simulink model "kadai2"  (R2024a)
settings: Solver=VariableStepAuto  StartTime=0.0  StopTime=10.0  RelTol=1e-3
values from neighbouring files (symbols this model uses):
  e0 = 24.6    [contstants.m]
  g = 9.8    [contstants.m]
  i0 = 1.21    [contstants.m]
  k = 2.9e-4    (= 0.00029)    [contstants.m]
  Ki = 2*k*i0/x0.^2    [contstants.m]
  Kx = 2*k*i0.^2/x0.^3    [contstants.m]
  L = 0.51    [contstants.m]
  M = 1.75    [contstants.m]
  R = 23.2    [contstants.m]
  s = tf('s')    [rlocus.m]
  x0 = 5.0e-3    (= 0.005)    [contstants.m]
libraries: slctrl_linear x2
settings Model: Creator=thistle  LastModifiedBy=thistle

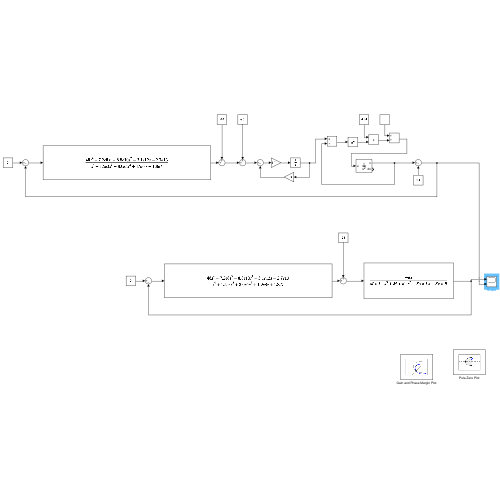
[thumbnail: Simulink's stored preview of the top-level diagram]
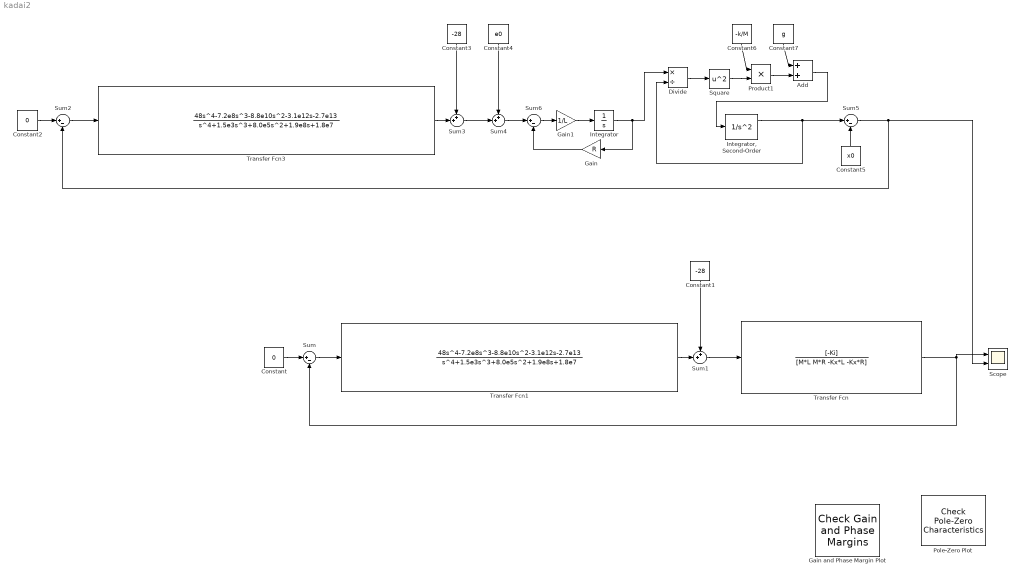
== system kadai2 ==
  Add : Sum
  Constant : Constant  Value=0
  Constant1 : Constant  Value=-28
  Constant2 : Constant  Value=0
  Constant3 : Constant  Value=-28
  Constant4 : Constant  Value=e0
  Constant5 : Constant  Value=x0
  Constant6 : Constant  Value=-k/M
  Constant7 : Constant  Value=g
  Divide : Product  Inputs=*/
  Gain : Gain  Gain=R
  Gain and Phase Margin Plot : slctrl_linear/Check Gain and Phase Margins  InstantiateOnLoad=on  SaveOperatingPoints=off  LinearizationIOs={'/Transfer Fcn', 1, 'out', 'on', '';'/Constant', 1, 'in', 'on', ''}  LinearizeAt=SnapshotTimes  SnapshotTimes=[0]  TriggerType=rising  SampleTime=auto  RateConversionMethod=zoh  PreWarpFreq=10  UseExactDelayModel=off  UseFullBlockNameLabels=off  UseBusSignalLabels=off  enabled=on  stopWhenAssertionFail=off  export=off  ViewDlgPos=[565.666666666667 151 510 390]  LaunchViewOnOpen=off  OpenViewOnLoad=off  FrequencyUnits=rad/s  MagnitudeUnits=dB  PhaseUnits=deg  TimeUnits=seconds  EnableMargins=off  GainMargin=[]  PhaseMargin=[]  PlotType=nyquist  FeedbackSign=-1
      settings: LibrarySourceBlock=slctrlblks/Linear Analysis Plots/Gain and Phase Margin Plot  SaveToWorkspace=off  SaveName=sys
  Gain1 : Gain  Gain=1/L
  Integrator : Integrator  InitialCondition=i0
  "Integrator, Second-Order" : SecondOrderIntegrator  ICX=x0
  Pole-Zero Plot : slctrl_linear/Check Pole-Zero Characteristics  InstantiateOnLoad=on  SaveOperatingPoints=off  LinearizationIOs={'/Constant', 1, 'in', 'on', '';'/Transfer Fcn', 1, 'out', 'on', ''}  LinearizeAt=SnapshotTimes  SnapshotTimes=[0]  TriggerType=rising  SampleTime=auto  RateConversionMethod=zoh  PreWarpFreq=10  UseExactDelayModel=off  UseFullBlockNameLabels=off  UseBusSignalLabels=off  enabled=on  stopWhenAssertionFail=off  export=off  ViewDlgPos=[1 1 1280 647.333333333333]  LaunchViewOnOpen=off  OpenViewOnLoad=off  FrequencyUnits=rad/s  MagnitudeUnits=dB  PhaseUnits=deg  TimeUnits=seconds  EnableSettlingTime=off  SettlingTime=[]  EnablePercentOvershoot=off  PercentOvershoot=[]  EnableDampingRatio=off  DampingRatio=[]  EnableNaturalFrequency=off  NaturalFrequencyBound=>=  NaturalFrequency=[]
      settings: LibrarySourceBlock=slctrlblks/Linear Analysis Plots/Pole-Zero Plot  SaveToWorkspace=off  SaveName=sys
  Product1 : Product
  Scope : Scope  NumInputPorts=2
  Square : Math  Operator=square
  Sum{,2,5..6} (4 alike) : Sum  Inputs=|+-
  Sum1 : Sum  Inputs=++|
  Sum3 : Sum  Inputs=++|
  Sum4 : Sum  Inputs=++|
  Transfer Fcn : TransferFcn  Numerator=[-Ki]  Denominator=[M*L M*R -Kx*L -Kx*R]
  Transfer Fcn1 : TransferFcn  Numerator=[48 -7.2e8 -8.8e10 -3.1e12 -2.7e13]  Denominator=[1 1.5e3 8.0e5 1.9e8 1.8e7]
  Transfer Fcn3 : TransferFcn  Numerator=[48 -7.2e8 -8.8e10 -3.1e12 -2.7e13]  Denominator=[1 1.5e3 8.0e5 1.9e8 1.8e7]
  wires:
  Constant/1 -> Sum/1
  Sum/1 -> Transfer Fcn1/1
  Transfer Fcn/1 -> Scope/1, Sum/2
  Transfer Fcn1/1 -> Sum1/2
  Sum1/1 -> Transfer Fcn/1
  Constant1/1 -> Sum1/1
  Square/1 -> Product1/2
  Sum3/1 -> Sum4/2
  Add/1 -> "Integrator, Second-Order"/1
  Constant4/1 -> Sum4/1
  Constant7/1 -> Add/1
  Constant6/1 -> Product1/1
  Sum5/1 -> Scope/2, Sum2/2
  Divide/1 -> Square/1
  Integrator/1 -> Gain/1, Divide/1
  Sum4/1 -> Sum6/1
  Constant2/1 -> Sum2/1
  Sum2/1 -> Transfer Fcn3/1
  Constant3/1 -> Sum3/1
  "Integrator, Second-Order"/1 -> Divide/2, Sum5/1
  Product1/1 -> Add/2
  Transfer Fcn3/1 -> Sum3/2
  Constant5/1 -> Sum5/2
  Gain/1 -> Sum6/2
  Sum6/1 -> Gain1/1
  Gain1/1 -> Integrator/1
